simulink subsystem "cart_pole_system_dynamics"  (R2023a)
settings: Solver=VariableStepAuto  StartTime=0.0  StopTime=10.0  RelTol=1e-3
undefined symbols (not defined in the file): g
settings Model: Creator=divij  LastModifiedBy=divij

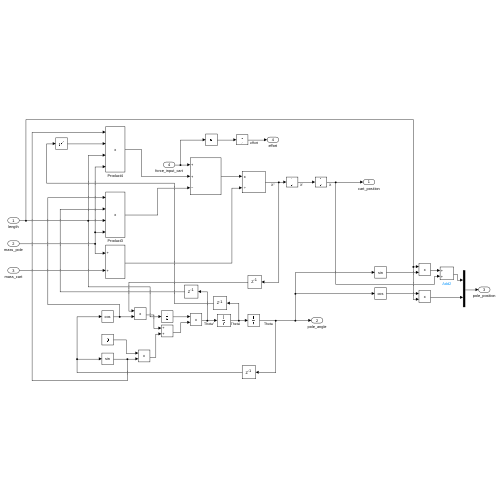
[thumbnail: Simulink's stored preview of the top-level diagram]
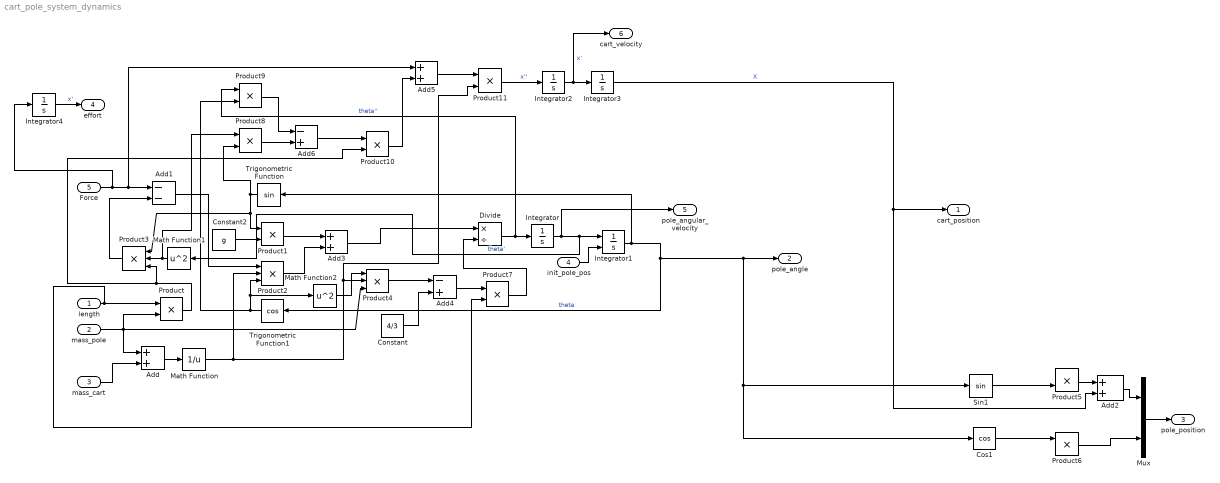
== system cart_pole_system_dynamics ==
  length : Inport
  mass_pole : Inport  Port=2
  mass_cart : Inport  Port=3
  init_pole_pos : Inport  Port=4
  Force : Inport  Port=5
  Add{,2..3,5} (4 alike) : Sum
  Add1 : Sum  Inputs=--
  Add4 : Sum  Inputs=-+
  Add6 : Sum  Inputs=-+
  Constant : Constant  Value=4/3
  Constant2 : Constant  Value=g
  Cos1 : Trigonometry  Operator=cos
  Divide : Product  Inputs=*/
  Integrator{,2..4} (4 alike) : Integrator
  Integrator1 : Integrator  InitialConditionSource=external
  Math Function : Math  Operator=reciprocal
  Math Function1 : Math  Operator=square
  Math Function2 : Math  Operator=square
  Mux : Mux  Inputs=2
  Product{,1,5..11} (9 alike) : Product
  Product2 : Product  Inputs=3
  Product3 : Product  Inputs=3
  Product4 : Product  Inputs=3
  Sin1 : Trigonometry
  Trigonometric Function : Trigonometry
  Trigonometric Function1 : Trigonometry  Operator=cos
  cart_position : Outport
  pole_angle : Outport  Port=2
  pole_position : Outport  Port=3
  effort : Outport  Port=4
  pole_angular_velocity : Outport  Port=5
  cart_velocity : Outport  Port=6
  wires:
  Integrator3/1 -> cart_position/1, Add2/2  "X"
  Sin1/1 -> Product5/2
  Cos1/1 -> Product6/1
  Product6/1 -> Mux/2
  Product5/1 -> Add2/1
  Add2/1 -> Mux/1
  Mux/1 -> pole_position/1
  mass_pole/1 -> Add/1, Product/2, Product4/3
  mass_cart/1 -> Add/2
  Add/1 -> Math Function/1
  Integrator/1 -> pole_angular_velocity/1, Integrator1/1, Math Function1/1  "theta'"
  Integrator1/1 -> Trigonometric Function1/1, pole_angle/1, Sin1/1, Cos1/1, Trigonometric Function/1  "theta"
  Constant2/1 -> Product1/2
  Trigonometric Function/1 -> Product8/2, Product1/1, Product3/1
  Math Function/1 -> Product2/2, Product4/2, Product11/2
  Force/1 -> Add1/1, Add5/1, Integrator4/1
  Math Function1/1 -> Product8/1, Product3/2
  Product3/1 -> Add1/2
  Add1/1 -> Product2/1
  Product1/1 -> Add3/1
  Product2/1 -> Add3/2
  Math Function2/1 -> Product4/1
  Product4/1 -> Add4/1
  Constant/1 -> Add4/2
  Add4/1 -> Product7/1
  length/1 -> Product7/2, Product/1
  Divide/1 -> Integrator/1, Product9/1  "theta''"
  Product7/1 -> Divide/2
  Add3/1 -> Divide/1
  init_pole_pos/1 -> Integrator1/2
  Product8/1 -> Add6/2
  Trigonometric Function1/1 -> Product2/3, Math Function2/1, Product9/2
  Product9/1 -> Add6/1
  Product/1 -> Product10/2, Product3/3
  Add6/1 -> Product10/1
  Product10/1 -> Add5/2
  Add5/1 -> Product11/1
  Product11/1 -> Integrator2/1  "x''"
  Integrator2/1 -> Integrator3/1, cart_velocity/1  "x'"
  Integrator4/1 -> effort/1  "x'"
